simulink model "B5G_SIM_PDR_ASH_V1"  (R2021a)
settings: Solver=ode4  StartTime=0.0  StopTime=dm.duration  FixedStep=dm.dt  RelTol=1e-3
InitFcn:
  | %b5g_init_param_sdr_v1;
StopFcn:
  | %b5g_post_param_sdr_v1;
  | 
  | %if mdl.OpenAfterSim.sdi
  | %   Simulink.sdi.view;
  | %end
  | 
  | %if mdl.OpenAfterSim.Scope
  | %   open_system(strcat(gcs,'/RateRwTorque'));
  | %end
model workspace (MAT data in the model file):
  RWModelType = 0
values from neighbouring files (symbols this model uses):
  dm = set_dm(dm)    [INIT_B5G_SIM_PDR_ASH.m]
  mdl = set_model_control()    [INIT_B5G_SIM_PDR_ASH.m]    (also in init_b5g_sim_pdr.m = set_model_control('B5G_SIM_PDR_V1'))
  rads2rpm = 60/(2*pi)    (= 9.54929658551)    [INIT_B5G_SIM_PDR_ASH.m]    (also in init_b5g_sim_pdr.m)
undefined symbols (not defined in the file or in its folder): Eclipse, fsw, MagSc, PVeci, Qi2b, RateSc, SunSc
libraries: vrlib x2, rptgenlib x1, aerolibtransform2 x1
(part 2 of 2)

== matlab function B5G_SIM_PDR_ASH_V1/Guidance & Control/ASH Mode/sun_sensor_contrl_processing/SunAngErr ==
  data: deltaAngle_c2b output; snr_fun input
function deltaAngle_c2b = RPLD_CTRL_PROC(snr_fun)

if ~snr_fun(4) 
    deltaAngle_c2b = [0;0;0];
    return;
end

vec_sun_b = snr_fun(1:3);
mag = norm(vec_sun_b);
if mag~=0
    vec_sun_b = vec_sun_b/mag;
end

%% DCM to Euler Angle Method
zb = (-1)*vec_sun_b';
yb = [0 vec_sun_b(3) -vec_sun_b(2)];
xb = cross(yb,zb);
R_B2C = [xb;yb;zb];

theta_c2b = -asin(R_B2C(3, 1));
phi_c2b = atan(R_B2C(3, 2) / R_B2C(3, 3));
% psi_c2b = atan2(R_B2C(2, 1), R_B2C(1, 1)); //3.14
psi_c2b = atan(R_B2C(2, 1) / R_B2C(1, 1));

%% deltaAngle_c2b = deltaAngle_b/c = -deltaAngle_c/b = -deltaAngle_b2c
deltaAngle_c2b = [phi_c2b; theta_c2b; psi_c2b];

== matlab function B5G_SIM_PDR_ASH_V1/Guidance & Control/ASH Mode/Subsystem/Variant Subsystem/BdotWithRate/MATLAB Function ==
  data: bdot_norm output; bdot input; Count_stab input; Stabilized input; Count_stab output; Stabilized output; fsw parameter
function [bdot_norm, Count_stab, Stabilized] = fcn(bdot,Count_stab, Stabilized, fsw)
    bdot_norm = norm(bdot);
    if Stabilized == 0
        if bdot_norm < fsw.ash_mgr.epsilon
            Count_stab = Count_stab + 1;
        else
            Count_stab = 0;
        end
        if Count_stab > fsw.ash_mgr.Tstab
            Stabilized = 1;
        end
    end

== matlab function B5G_SIM_PDR_ASH_V1/Guidance & Control/ASH Mode/Subsystem/Variant Subsystem/BdotWithRate/BdotWithRate ==
  settings: updateMethod=DISCRETE
  data: Bb input; Mc output size=3; fsw parameter; bdot output size=3; RateSc input
%% BdotControl
function [Mc,bdot] = Bdot2(Bb, fsw, RateSc)

Bdot= -cross(RateSc,Bb);
nBdot= norm(Bdot);

%% divided-by-zero check
if abs(nBdot-eps)> 1e-10
    bdot= Bdot/norm(Bb); %% Correction: Fix Tutorial Typo
else
    bdot= zeros(3,1);
end

Mc = -fsw.wXbdot_gain .* bdot;

end

== matlab function B5G_SIM_PDR_ASH_V1/Space Environment Models/Orbit Propagator /J2 Ben ==
  data: X input; Xdot output; dm parameter
function Xdot = J2(X, dm)

r = X(1:3);
v = X(4:6);
J2 = 0.484165143790815D-03*(5)^0.5;
GMe = 3.986004418e14;                % m^3*s^-2
Re = 6378137;                        % earth radius, m
k_1_2 = -GMe/norm(r)^3 * (1+ 1.5 *J2* (Re/norm(r))^2 * (1 - 5* (r(3)/norm(r))^2) );
k_3 = -GMe/norm(r)^3 * (1+ 1.5 *J2* (Re/norm(r))^2 * (3 - 5* (r(3)/norm(r))^2) );
a = [k_1_2*r(1); k_1_2*r(2); k_3*r(3)];
Xdot=[v; a];

% Re   = 6378137.00;%m
% mu_e = 3.986004418e14;%3.986004418e14;
% 
% p = X(1:3);
% v = X(4:6);
% R = norm(p);
% 
% 
% J2 = 0.001082626173852;%0.001082626173852;% C20_bar = -0.484165143790815D-03 from EGM2008
% %0.001082626683553151; STK
%      
% ReOverR_2 = (Re/R)^2;
% sinphi_2   = (p(3)/R)^2;
% muOverR_3 = mu_e/R^3;
% vdot=[-muOverR_3*(1+1.5*J2*ReOverR_2*(1-5*sinphi_2));...
%       -muOverR_3*(1+1.5*J2*ReOverR_2*(1-5*sinphi_2));...
%       -muOverR_3*(1+1.5*J2*ReOverR_2*(3-5*sinphi_2))].*p;
%      
% Xdot=[v; vdot];

== matlab function B5G_SIM_PDR_ASH_V1/Space Environment Models/Orbit Propagator /J2 Jack ==
  data: X input; Xdot output; dm parameter
function Xdot = J2(X, dm)

Re   = 6378137.00;%m
mu_e = 3.986004418e14;%3.986004418e14;

p = X(1:3);
v = X(4:6);
R = norm(p);


J2 = 0.001082626173852;%0.001082626173852;% C20_bar = -0.484165143790815D-03 from EGM2008
%0.001082626683553151; STK
     
ReOverR_2 = (Re/R)^2;
sinphi_2   = (p(3)/R)^2;
muOverR_3 = mu_e/R^3;
vdot=[-muOverR_3*(1+1.5*J2*ReOverR_2*(1-5*sinphi_2));...
      -muOverR_3*(1+1.5*J2*ReOverR_2*(1-5*sinphi_2));...
      -muOverR_3*(1+1.5*J2*ReOverR_2*(3-5*sinphi_2))].*p;
     
Xdot=[v; vdot];

== matlab function B5G_SIM_PDR_ASH_V1/RWA/Nonlinear/RW1/MATLAB Function ==
  data: torque input; torque output; rate input; dm parameter
function torque = torqueBox(torque,rate, dm)

momentum = dm.rw_mdl.moi * rate;
maxAngMom = dm.rw_mdl.maxAngMom;
AvlAngMom = dm.rw_mdl.avlAngMom;
maxTorque = dm.rw_mdl.maxTorque;

if momentum >= AvlAngMom && momentum <= maxAngMom
    torque = 1 + (-maxTorque) * (momentum);
elseif momentum <= -AvlAngMom && momentum >= (-maxAngMom)
    torque = -1 + (-maxTorque) * (momentum);
end

== matlab function B5G_SIM_PDR_ASH_V1/RWA/Nonlinear/RW2/MATLAB Function ==
  data: torque input; torque output; rate input; dm parameter
function torque = torqueBox(torque,rate, dm)

momentum = dm.rw_mdl.moi * rate;
maxAngMom = dm.rw_mdl.maxAngMom;
AvlAngMom = dm.rw_mdl.avlAngMom;
maxTorque = dm.rw_mdl.maxTorque;

if momentum >= AvlAngMom && momentum <= maxAngMom
    torque = 1 + (-maxTorque) * (momentum);
elseif momentum <= -AvlAngMom && momentum >= (-maxAngMom)
    torque = -1 + (-maxTorque) * (momentum);
end

== matlab function B5G_SIM_PDR_ASH_V1/Space Environment Models/Orbit Propagator /gravityField/TwoBodyRHS/MATLAB Function ==
  data: X input; Xdot output; dm parameter
function Xdot = TwoBodyRHS(X, dm)

r = X(1:3);
v = X(4:6);
Xdot=[v; -(dm.mu_e*r/norm(r)^3)];

== matlab function B5G_SIM_PDR_ASH_V1/Space Environment Models/Orbit Propagator /gravityField/J2/J2 Jack ==
  data: X input; Xdot output; dm parameter
function Xdot = J2(X, dm)

Re   = 6378137.00;%m
mu_e = 3.986004418e14;%3.986004418e14;

p = X(1:3);
v = X(4:6);
R = norm(p);


J2 = 0.001082626173852;%0.001082626173852;% C20_bar = -0.484165143790815D-03 from EGM2008
%0.001082626683553151; STK
     
ReOverR_2 = (Re/R)^2;
sinphi_2   = (p(3)/R)^2;
muOverR_3 = mu_e/R^3;
vdot=[-muOverR_3*(1+1.5*J2*ReOverR_2*(1-5*sinphi_2));...
      -muOverR_3*(1+1.5*J2*ReOverR_2*(1-5*sinphi_2));...
      -muOverR_3*(1+1.5*J2*ReOverR_2*(3-5*sinphi_2))].*p;
     
Xdot=[v; vdot];

== matlab function B5G_SIM_PDR_ASH_V1/RWA/Nonlinear/RW3/MATLAB Function ==
  data: torque input; torque output; rate input; dm parameter
function torque = torqueBox(torque,rate, dm)

momentum = dm.rw_mdl.moi * rate;
maxAngMom = dm.rw_mdl.maxAngMom;
AvlAngMom = dm.rw_mdl.avlAngMom;
maxTorque = dm.rw_mdl.maxTorque;

if momentum >= AvlAngMom && momentum <= maxAngMom
    torque = 1 + (-maxTorque) * (momentum);
elseif momentum <= -AvlAngMom && momentum >= (-maxAngMom)
    torque = -1 + (-maxTorque) * (momentum);
end

== matlab function B5G_SIM_PDR_ASH_V1/RWA/Nonlinear/RW4/MATLAB Function ==
  data: torque input; torque output; rate input; dm parameter
function torque = torqueBox(torque,rate, dm)

momentum = dm.rw_mdl.moi * rate;
maxAngMom = dm.rw_mdl.maxAngMom;
AvlAngMom = dm.rw_mdl.avlAngMom;
maxTorque = dm.rw_mdl.maxTorque;

if momentum >= AvlAngMom && momentum <= maxAngMom
    torque = 1 + (-maxTorque) * (momentum);
elseif momentum <= -AvlAngMom && momentum >= (-maxAngMom)
    torque = -1 + (-maxTorque) * (momentum);
end
